simulink model "Inner_Loop_Linear_DCM"  (R2024b)
settings: Solver=ode15s  StartTime=0.0  StopTime=0.1  RelTol=1e-6  AbsTol=1e-8
undefined symbols (not defined in the file or in its folder): Ci, ctrl, DiscIntNeverNeededParam, i_start, i_stop, Ts
libraries: cstblocks x2
settings Model: SimulationMode=accelerator  Creator=rs  LastModifiedBy=overflow
settings SolverCC: AutoScaleAbsTol=off  ZeroCrossAlgorithm=Adaptive  AlgebraicLoopSolver=TrustRegion
settings DataIOCC: SaveFormat=Array  SaveOutput=off  SignalLogging=off  DSMLogging=off  SaveTime=off  ReturnWorkspaceOutputs=off  TimeSaveName=t  OutputSaveName=y
settings DebuggingCC: UnconnectedInputMsg=warning  UnconnectedOutputMsg=warning  UnconnectedLineMsg=warning  ArithmeticOperatorsInVariantConditions=warning
settings ModelReferenceCC: EnableRefExpFcnMdlSchedulingChecks=on
settings SFSimCC: SimUseLocalCustomCode=off  CustomCodeUndefinedFunction=UseInterfaceOnly
settings RTWCC: RTWUseLocalCustomCode=off  GPUComputeCapability=3.5

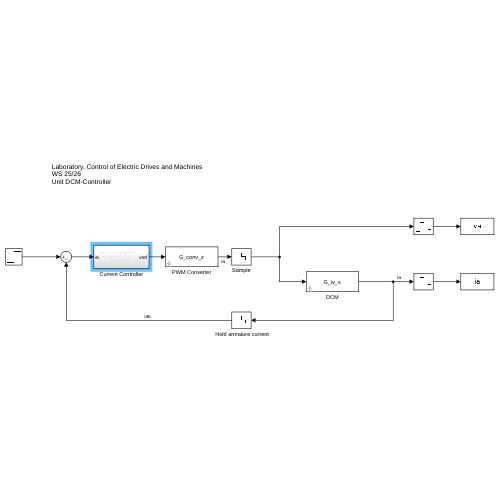
[thumbnail: Simulink's stored preview of the top-level diagram]
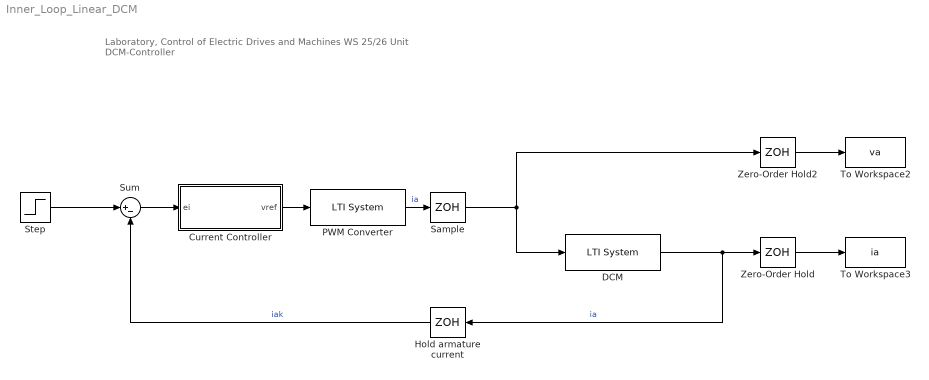
== system Inner_Loop_Linear_DCM ==
  note: Laboratory, Control of Electric Drives and Machines
      | WS 25/26
      | Unit DCM-Controller
  " Hold armature current" : ZeroOrderHold  SampleTime=-1
  Current Controller : Subsystem
  DCM : cstblocks/LTI System  sys=G_iv_s  IC=[]  PadeOrder=0
  PWM Converter : cstblocks/LTI System  sys=G_conv_z  IC=[]  PadeOrder=0
  Sample : ZeroOrderHold  SampleTime=-1
  Step : Step  Time=0.05  Before=i_start  After=i_stop  SampleTime=0
  Sum : Sum  Inputs=|+-
  To Workspace2 : ToWorkspace  VariableName=va  SaveFormat=Timeseries  SampleTime=-1
  To Workspace3 : ToWorkspace  VariableName=ia  SaveFormat=Timeseries  SampleTime=-1
  Zero-Order Hold : ZeroOrderHold  SampleTime=Ts
  Zero-Order Hold2 : ZeroOrderHold  SampleTime=Ts
  wires:
  Zero-Order Hold/1 -> To Workspace3/1
  DCM/1 -> Zero-Order Hold/1, " Hold armature current"/1  "ia"
  Zero-Order Hold2/1 -> To Workspace2/1
  Sum/1 -> Current Controller/1(ei)
  " Hold armature current"/1 -> Sum/2  "iak"
  Step/1 -> Sum/1
  Sample/1 -> DCM/1, Zero-Order Hold2/1
  PWM Converter/1 -> Sample/1  "ia"
  Current Controller/1(vref) -> PWM Converter/1

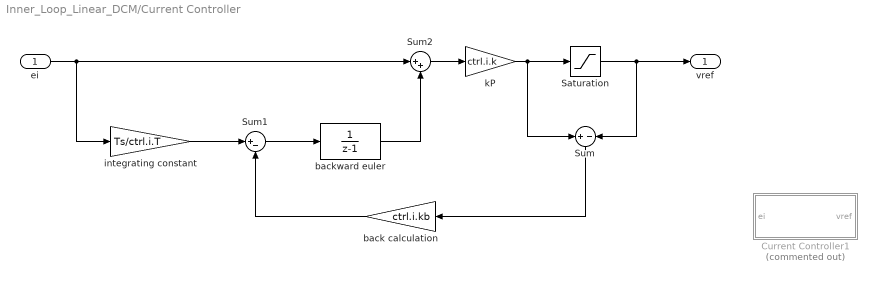
== system Inner_Loop_Linear_DCM/Current Controller ==
  ei : Inport
  Current Controller1 : Subsystem  Commented=on
  Saturation : Saturate  UpperLimit=ctrl.i.satP  LowerLimit=ctrl.i.satN
  Sum : Sum  Inputs=+|-
  Sum1 : Sum  Inputs=|+-
  Sum2 : Sum  Inputs=|++
  back calculation : Gain  Gain=ctrl.i.kb
  backward euler : DiscreteTransferFcn  Denominator=[1 -1]  InitialStates=i_start
  integrating constant : Gain  Gain=Ts/ctrl.i.T
  kP : Gain  Gain=ctrl.i.k
  vref : Outport
  wires:
  Sum1/1 -> backward euler/1
  integrating constant/1 -> Sum1/1
  Saturation/1 -> vref/1, Sum/2
  Sum/1 -> back calculation/1
  back calculation/1 -> Sum1/2
  ei/1 -> integrating constant/1, Sum2/1
  Sum2/1 -> kP/1
  kP/1 -> Sum/1, Saturation/1
  backward euler/1 -> Sum2/2

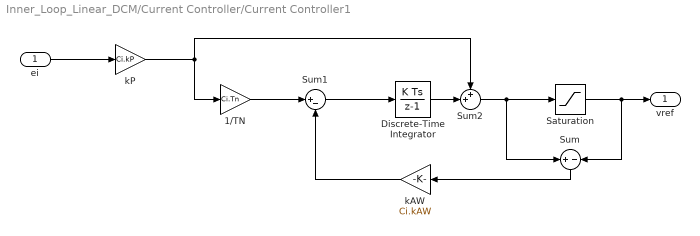
== system Inner_Loop_Linear_DCM/Current Controller/Current Controller1 ==
  ei : Inport
  1/TN : Gain  Gain=Ci.Tn
  Discrete-Time Integrator : DiscreteIntegrator  SampleTime=-1  ICPrevOutput=DiscIntNeverNeededParam  ICPrevScaledInput=DiscIntNeverNeededParam
  Saturation : Saturate
  Sum : Sum  Inputs=+|-
  Sum1 : Sum  Inputs=|+-
  Sum2 : Sum  Inputs=++|
  kAW : Gain  Gain=Ci.kAW
  kP : Gain  Gain=Ci.kP
  vref : Outport
  wires:
  Sum1/1 -> Discrete-Time Integrator/1
  1/TN/1 -> Sum1/1
  Discrete-Time Integrator/1 -> Sum2/2
  ei/1 -> kP/1
  Sum2/1 -> Sum/1, Saturation/1
  Saturation/1 -> Sum/2, vref/1
  Sum/1 -> kAW/1
  kAW/1 -> Sum1/2
  kP/1 -> Sum2/1, 1/TN/1
